simulink model "PitchSys"  (R2024b)
settings: Solver=ode1  StartTime=0.00  StopTime=10.00  FixedStep=0.01  RelTol=1e-3  EnableMultiTasking=on
undefined symbols (not defined in the file or in its folder): Jp, k_d, k_s, l2
settings Model: Creator=bjones  LastModifiedBy=leeta
settings SolverCC: AlgebraicLoopSolver=TrustRegion
settings DataIOCC: SaveFormat=Array  SignalLoggingSaveFormat=ModelDataLogs  ReturnWorkspaceOutputs=off
settings OptimizationCC: BlockReduction=off  BooleanDataType=off  ExpressionDepthLimit=2147483647  LifeSpan=inf
settings DebuggingCC: SaveWithParameterizedLinksMsg=none  UnderspecifiedInitializationDetection=Classic  MergeDetectMultiDrivingBlocksExec=none  SignalResolutionControl=TryResolveAllWithWarning  MultiTaskDSMMsg=warning  MultiTaskCondExecSysMsg=none  FcnCallInpInsideContextMsg=warning  UnconnectedInputMsg=warning  UnconnectedOutputMsg=warning  UnconnectedLineMsg=warning  StateNameClashWarn=warning  SFUnexpectedBacktrackingDiag=warning  SFNoUnconditionalDefaultTransitionDiag=warning  SFExecutionAtInitializationDiag=none  ArithmeticOperatorsInVariantConditions=warning
settings HardwareCC: ProdBitPerPointer=32  ProdBitPerSizeT=32  ProdBitPerPtrDiffT=32  ProdLargestAtomicFloat=None  ProdIntDivRoundTo=Undefined  ProdEndianess=Unspecified  ProdWordSize=32  ProdHWDeviceType=32-bit Generic  TargetBitPerPointer=64  TargetBitPerSizeT=64  TargetBitPerPtrDiffT=64  TargetLongLongMode=on  TargetIntDivRoundTo=Zero  TargetEndianess=LittleEndian  TargetWordSize=64  TargetHWDeviceType=MATLAB Host  ProdEqTarget=off
settings ModelReferenceCC: EnableRefExpFcnMdlSchedulingChecks=on  PropagateSignalLabelsOutOfModel=off
settings SFSimCC: SimUseLocalCustomCode=off  CustomCodeUndefinedFunction=UseInterfaceOnly
settings RTWCC: RTWUseLocalCustomCode=off  GPUComputeCapability=3.5
settings CodeAppCC: StateflowObjectComments=on
settings GRTTargetCC: TargetLangStandard=C89/C90 (ANSI)  CombineOutputUpdateFcns=off  GRTInterface=on
settings ConfigComp: CovMetricSettings=dw  CovSaveCumulativeToWorkspaceVar=on  CovSaveSingleToWorkspaceVar=on  CovExternalEMLEnable=off  CovSFcnEnable=off

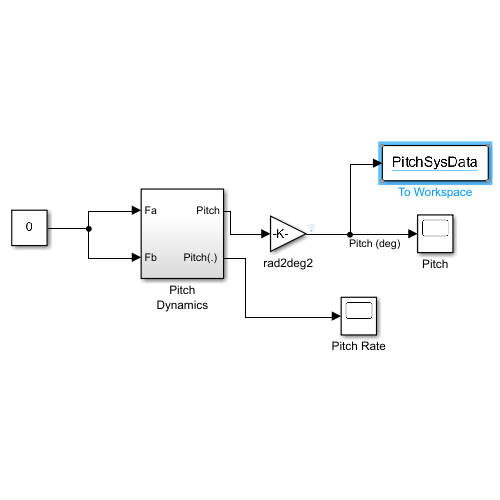
[thumbnail: Simulink's stored preview of the top-level diagram]
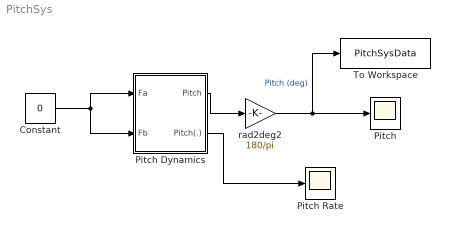
== system PitchSys ==
  Constant : Constant  Value=0
  Pitch : Scope
  Pitch Dynamics : Subsystem
  Pitch Rate : Scope
  To Workspace : ToWorkspace  VariableName=PitchSysData  SaveFormat=Timeseries  SampleTime=-1
  rad2deg2 : Gain  Gain=180/pi  SaturateOnIntegerOverflow=on  OutDataTypeStr=Inherit: Same as input  ParamDataTypeStr=Inherit: Same as input
  wires:
  Pitch Dynamics/1(Pitch) -> rad2deg2/1
  rad2deg2/1 -> To Workspace/1, Pitch/1  "Pitch (deg)"
  Constant/1 -> Pitch Dynamics/1(Fa), Pitch Dynamics/2(Fb)
  Pitch Dynamics/2("Pitch(.) ") -> Pitch Rate/1

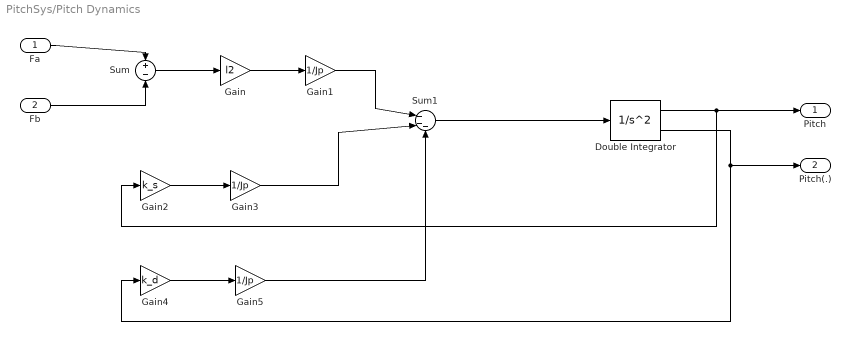
== system PitchSys/Pitch Dynamics ==
  Fa : Inport
  Fb : Inport  Port=2
  Double Integrator : SecondOrderIntegrator  ICX=p0  LimitX=on  UpperLimitX=p_lim_u  LowerLimitX=p_lim_l
  Gain : Gain  Gain=l2
  Gain1 : Gain  Gain=1/Jp
  Gain2 : Gain  Gain=k_s
  Gain3 : Gain  Gain=1/Jp
  Gain4 : Gain  Gain=k_d
  Gain5 : Gain  Gain=1/Jp
  Sum : Sum  Inputs=+-
  Sum1 : Sum  Inputs=|---
  Pitch : Outport
  "Pitch(.) " : Outport  Port=2
  wires:
  Double Integrator/1 -> Gain2/1, Pitch/1
  Fa/1 -> Sum/1
  Fb/1 -> Sum/2
  Sum/1 -> Gain/1
  Gain/1 -> Gain1/1
  Gain1/1 -> Sum1/1
  Gain2/1 -> Gain3/1
  Gain3/1 -> Sum1/2
  Gain4/1 -> Gain5/1
  Gain5/1 -> Sum1/3
  Sum1/1 -> Double Integrator/1
  Double Integrator/2 -> "Pitch(.) "/1, Gain4/1
